simulink model "Speedgoat"  (R2023b)
settings: Solver=FixedStepDiscrete  StartTime=0.0  StopTime=1000000000  FixedStep=0.001  RelTol=1e-3  EnableMultiTasking=on
undefined symbols (not defined in the file): IO397
libraries: speedgoatlib_fpga_analog_io x2, speedgoatlib_fpga_dio x1, speedgoatlib_fpga x1
settings Model: Creator=yaman  LastModifiedBy=oliver
settings SolverCC: ConcurrentTasks=on  AlgebraicLoopSolver=TrustRegion  PositivePriorityOrder=on  InsertRTBMode=Never (minimum delay)
settings DataIOCC: SaveFormat=Array  SaveState=on  SignalLoggingName=logsOut
settings OptimizationCC: BlockReduction=off  BooleanDataType=off  OptimizeBlockIOStorage=off  BufferReuse=off  ReuseModelBlockBuffer=off  GlobalBufferReuse=off  ExpressionFolding=off  LocalBlockOutputs=off  InitFltsAndDblsToZero=on  OptimizeDataStoreBuffers=off  BusAssignmentInplaceUpdate=off
settings DebuggingCC: SaveWithParameterizedLinksMsg=none  UnderspecifiedInitializationDetection=Classic  MergeDetectMultiDrivingBlocksExec=none  CheckExecutionContextPreStartOutputMsg=on  SignalResolutionControl=TryResolveAllWithWarning  TasksWithSamePriorityMsg=none  UnconnectedInputMsg=warning  UnconnectedOutputMsg=warning  UnconnectedLineMsg=warning  SFUnexpectedBacktrackingDiag=warning  SFNoUnconditionalDefaultTransitionDiag=warning  SFExecutionAtInitializationDiag=none  ArithmeticOperatorsInVariantConditions=warning
settings HardwareCC: ProdBitPerLong=64  ProdLongLongMode=on  ProdHWDeviceType=Intel->x86-64 (Linux 64)
settings ModelReferenceCC: EnableRefExpFcnMdlSchedulingChecks=on  PropagateSignalLabelsOutOfModel=off
settings SFSimCC: SimUseLocalCustomCode=off  SimTargetLang=C++
settings RTWCC: Description=Simulink Real-Time  SystemTargetFile=slrealtime.tlc  TemplateMakefile=slrealtime_default_tmf  RTWUseLocalCustomCode=off  Toolchain=Simulink Real-Time Toolchain  BuildConfiguration=Faster Runs  CodeExecutionProfiling=on  TargetLang=C++  DLArmComputeVersion=19.05
settings CodeAppCC: StateflowObjectComments=on
settings SimulinkRealTimeTargetCC: MATLABClassNameForMDSCustomization=Simulink.SoftwareTarget.GRTCustomization  UseGCCFastMath=on
settings ConfigComp: CovMetricSettings=dw  CovSaveCumulativeToWorkspaceVar=on  CovSaveSingleToWorkspaceVar=on  CovExternalEMLEnable=off  CovSFcnEnable=off

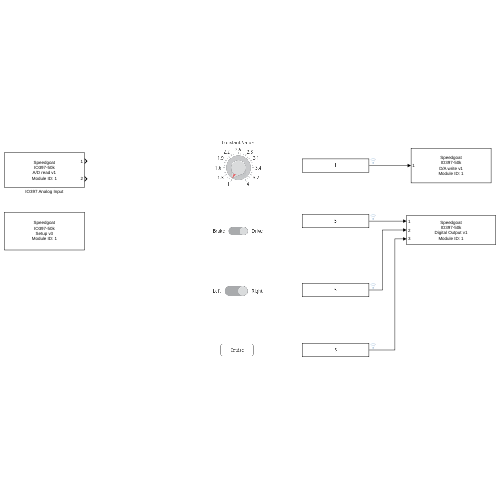
[thumbnail: Simulink's stored preview of the top-level diagram]
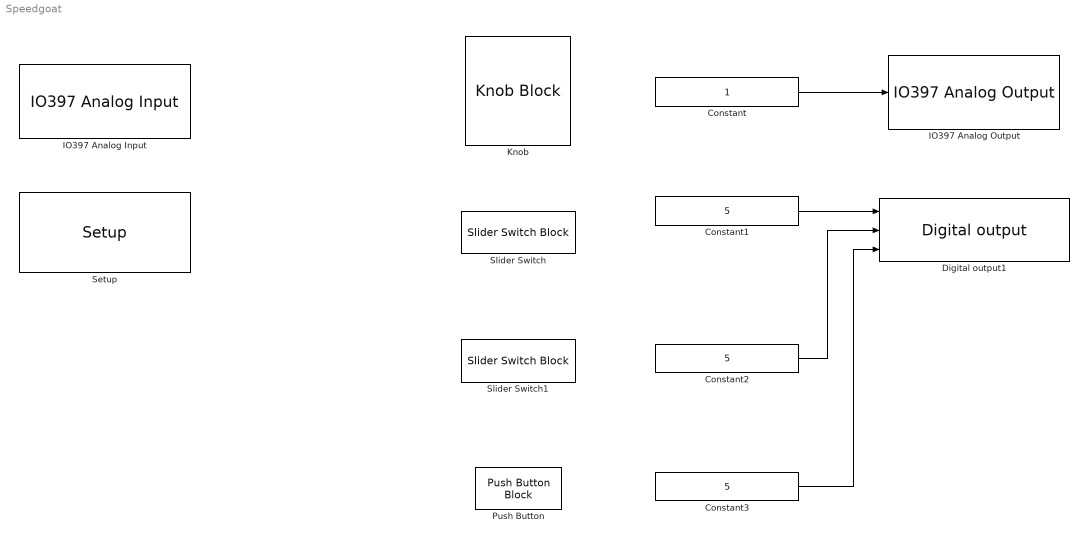
== system Speedgoat ==
  Constant : Constant  OutMin=[0]  OutMax=[5]
  Constant1 : Constant  Value=5  OutMin=[0]  OutMax=[5]
  Constant2 : Constant  Value=5  OutMin=[0]  OutMax=[5]
  Constant3 : Constant  Value=5  OutMin=[0]  OutMax=[5]
  Digital output1 : speedgoatlib_fpga_dio/Digital output  id=1  chan=[1 2 3]  init=[0]  reset=[0]  ts=0.001  vectorizeInput=off
      settings: SourceProductName=Simulink Real-Time: Speedgoat I/O Blockset
  IO397 Analog Input : speedgoatlib_fpga_analog_io/IO397 Analog Input  openMaskCallback=0  id=1  chan=[1 2]  range=+5.12 V  parAiTriggerMode=I/O Module Clock  parAiInternalSignal=None  parAiDioTriggerChannel=1  parAiSampleRate=0  trigger=Initiator  ts=0.001
      settings: SourceProductName=Simulink Real-Time: Speedgoat I/O Blockset
  IO397 Analog Output : speedgoatlib_fpga_analog_io/IO397 Analog Output  id=1  chan=[1]  initVal=0  resetVal=0  ts=0.001  span=+5 V
      settings: SourceProductName=Simulink Real-Time: Speedgoat I/O Blockset
  Knob : KnobBlock  ScaleMin=1  ScaleMax=4
  Push Button : PushButtonBlock  ButtonText=Cruise  OnValue=0  OffValue=5.000000
  Setup : speedgoatlib_fpga/Setup/Setup  board=IO397-50k  id=1  device_id=1  frontIO=None  rearIO=None  bitstreamFile=speedgoat_IO397_HIL.mat  rev=7.000000  timestamp_string=11/03/24 17:21:57  fpgaFreq=75 MHz  fpgaTick=13.33 ns  ProgSpiFlash=off  ProgBPIFlash=off  pciSlot=-1  useFpgaDmaController=off  PullRPort0=pull-up 3.3V  VioPort0=3.3V  PullRPort1=pull-up 3.3V  VioPort1=3.3V  PullRPort2=pull-up 3.3V  VioPort2=3.3V  PullRPort3=pull-up 3.3V  VioPort3=3.3V  PullRPort4=pull-up 3.3V  VioPort4=3.3V  PullRPort5=pull-up 3.3V  VioPort5=3.3V  PullRPort6=pull-up 3.3V  VioPort6=3.3V  diffLineTermination_rear1=on  diffLineTermination_rear2=on  diffLineTermination_rear3=on  diffLineTermination_rear4=on  diffLineTermination_rear5=on  diffLineTermination_rear6=on  diffLineTermination_rear7=on  diffLineTermination_rear8=on  PullRPort15=weak pull-up 5.0V  PullRPort31=pull-up 3.3V  PullRPort47=pull-up 3.3V  PullRPort63=pull-up 3.3V  diffLineTermination_1=on  diffLineTermination_2=on  diffLineTermination_3=on  diffLineTermination_4=on  diffLineTermination_5=on  diffLineTermination_6=on  diffLineTermination_7=on  diffLineTermination_8=on  diffLineTermination_9=on  diffLineTermination_10=on  diffLineTermination_11=on  diffLineTermination_12=on  diffLineTermination_13=on  diffLineTermination_14=on  diffLineTermination_15=on  diffLineTermination_16=on  diffLineTermination_17=on  diffLineTermination_18=on  diffLineTermination_19=on  diffLineTermination_20=on  diffLineTermination_21=on  diffLineTermination_22=on  diffLineTermination_23=on  diffLineTermination_24=on  diffLineTermination_25=on  diffLineTermination_26=on  diffLineTermination_27=on  diffLineTermination_28=on  diffLineTermination_29=on  diffLineTermination_30=on  diffLineTermination_31=on  diffLineTermination_32=on  Vo_36x_1=3.3V  Vi_Pull_36x_1=Floating  Vo_36x_2=3.3V  Vi_Pull_36x_2=Floating  Vo_36x_3=3.3V  Vi_Pull_36x_3=Floating  Vo_36x_4=3.3V  Vi_Pull_36x_4=Floating  Vo_36x_5=3.3V  Vi_Pull_36x_5=Floating  Vo_36x_6=3.3V  Vi_Pull_36x_6=Floating  Vo_36x_7=3.3V  Vi_Pull_36x_7=Floating  Vo_36x_8=3.3V  Vi_Pull_36x_8=Floating  Vo_36x_9_16=3.3V  Vi_Pull_36x_9_16=Floating  Vo_36x_17_24=3.3V  Vi_Pull_36x_17_24=Floating  Vo_36x_25_32=3.3V  Vi_Pull_36x_25_32=Floating  Vo_36x_33_40=3.3V  Vi_Pull_36x_33_40=Floating  Vo_36x_41_48=3.3V  Vi_Pull_36x_41_48=Floating  Vo_36x_49_56=3.3V  Vi_Pull_36x_49_56=Floating  Vo_36x_57_64=3.3V  Vi_Pull_36x_57_64=Floating
      settings: SourceProductName=Simulink Real-Time: Speedgoat I/O Blockset
  Slider Switch : SliderSwitchBlock  LabelPosition=Hide
      settings: Values={{'Brake', 'Drive'}, [0.5 5]}
  Slider Switch1 : SliderSwitchBlock  LabelPosition=Hide
      settings: Values={{'Left', 'Right'}, [0 5]}
  wires:
  Constant1/1 -> Digital output1/1
  Constant/1 -> IO397 Analog Output/1
  Constant2/1 -> Digital output1/2
  Constant3/1 -> Digital output1/3
